simulink model "TeamA_PAsqualo1"  (R2020a)
settings: Solver=VariableStepAuto  StartTime=0.0  StopTime=stop_time  FixedStep=0.05  RelTol=1e-3
InitFcn:
  | main_init
values from neighbouring files (symbols this model uses):
  a1 = rho * D^4 * alpha1    (= 0.000388302366464)    [data_current.m]    (also in main_init.m)
  a2 = -rho * D^3 * alpha2 * (1 - omega)    (= 0.0037030698432)    [data_current.m]    (also in main_init.m)
  ag = [Ax Ay Az]'    [init_modello.m]
  alpha1 = 0.0113    [data_current.m]    (also in main_init.m)
  alpha2 = -0.0091    [data_current.m]    (also in main_init.m)
  areaOfInterestCorner = [42.317744;10.915136; 0]    [init_controllo.m]    (also in missionA.m = [42.317744)
  bg = [Bx By Bz]'    [init_modello.m]
  cd_pitch = 0.7    [init_modello.m]
  cd_roll = 0.04    [init_modello.m]
  cd_x = 0.4    [init_modello.m]
  cd_y = 1    [init_modello.m]
  cd_yaw = 0.7    [init_modello.m]
  cd_z = 1    [init_modello.m]
  cg = [Cx Cy Cz]'    [init_modello.m]
  D = 0.076    [data_current.m]    (also in main_init.m)
  dead_zone_limit = 31.5    [data_current.m]    (also in main_init.m)
  dg = [Dx Dy Dz]'    [init_modello.m]
  eg = [Ex Ey Ez]'    [init_modello.m]
  fg = [Fx Fy Fz]'    [init_modello.m]
  g = 9.81    [init_modello.m]
  galleggiamento = 66.5386    [init_controllo.m]
  gg = [Gx Gy Gz]'    [init_modello.m]
  H0 = 0    [init_modello.m]
  init_position = [pointP(1),pointP(2),0.15,0,0,deg2rad(angle)]'    [appunti.m]    (also in init_modello.m = [pointP(1),pointP(2),0.15,0,0,deg2rad(alpha)]')
  init_velocity = [0 0 0 0 0 0]'    [init_modello.m]
  initial_state_cov = blkdiag(diag(cov_gps(1,1:2)), cov_depth*eye(n_state_filter-2))    [init_navigazione.m]
  Ixx = 0.93304097392    [init_modello.m]
  Ixy = 0    [init_modello.m]
  Ixz = 0    [init_modello.m]
  Iyy = 25.58745481378    (= 25.5874548138)    [init_modello.m]
  Iyz = 0    [init_modello.m]
  Izz = 25.58745481378    (= 25.5874548138)    [init_modello.m]
  K_i_heave_div = 20    [init_controllo.m]
  K_i_heave_pos = 1    [init_controllo.m]
  K_i_heave_surf = 20    [init_controllo.m]
  K_i_heave_trans = 5    [init_controllo.m]
  K_i_heave_turn = 5    [init_controllo.m]
  K_i_pitch_div = 0    [init_controllo.m]
  K_i_pitch_pos = 0.1*0    (= 0)    [init_controllo.m]
  K_i_pitch_surf = 0    [init_controllo.m]
  K_i_pitch_trans = 0    [init_controllo.m]
  K_i_pitch_turn = 0    [init_controllo.m]
  K_i_roll_div = 0    [init_controllo.m]
  K_i_roll_pos = 0.1*0    (= 0)    [init_controllo.m]
  K_i_roll_surf = 1    [init_controllo.m]
  K_i_roll_trans = 0    [init_controllo.m]
  K_i_roll_turn = 0    [init_controllo.m]
  K_i_surge_div = 3    [init_controllo.m]
  K_i_surge_pos = 0.1679*30    (= 5.037)    [init_controllo.m]
  K_i_surge_surf = 3    [init_controllo.m]
  K_i_surge_trans = 0.1679*15    (= 2.5185)    [init_controllo.m]
  K_i_surge_turn = 0.1679*60    (= 10.074)    [init_controllo.m]
  K_i_sway_div = 6    [init_controllo.m]
  K_i_sway_pos = 5    [init_controllo.m]
  K_i_sway_surf = 3    [init_controllo.m]
  K_i_sway_trans = 2    [init_controllo.m]
  K_i_sway_turn = 50    [init_controllo.m]
  K_i_yaw_div = 0    [init_controllo.m]
  K_i_yaw_pos = 1    [init_controllo.m]
  K_i_yaw_surf = 0    [init_controllo.m]
  K_i_yaw_trans = 20    [init_controllo.m]
  K_i_yaw_turn = 3    [init_controllo.m]
  K_p_heave_div = 200    [init_controllo.m]
  K_p_heave_pos = 320    [init_controllo.m]
  K_p_heave_surf = 200    [init_controllo.m]
  K_p_heave_trans = 170    [init_controllo.m]
  K_p_heave_turn = 170    [init_controllo.m]
  K_p_phi_div = 0.15    [init_controllo.m]
  K_p_phi_pos = 1*0.1    (= 0.1)    [init_controllo.m]
  K_p_phi_surf = 0.15    [init_controllo.m]
  K_p_phi_trans = 0.1    [init_controllo.m]
  K_p_phi_turn = 0.1    [init_controllo.m]
  K_p_pitch_div = 50    [init_controllo.m]
  K_p_pitch_pos = 25    [init_controllo.m]
  K_p_pitch_surf = 50    [init_controllo.m]
  K_p_pitch_trans = 25    [init_controllo.m]
  K_p_pitch_turn = 25    [init_controllo.m]
  K_p_psi_div = 0.3    [init_controllo.m]
  K_p_psi_pos = 0.25    [init_controllo.m]
  K_p_psi_surf = 0.3    [init_controllo.m]
  K_p_psi_trans = 0.2    [init_controllo.m]
  K_p_roll_div = 10    [init_controllo.m]
  K_p_roll_pos = 0.1*40    (= 4)    [init_controllo.m]
  K_p_roll_surf = 10    [init_controllo.m]
  K_p_roll_trans = 0.1*40    (= 4)    [init_controllo.m]
  K_p_roll_turn = 4    [init_controllo.m]
  K_p_surge_div = 80    [init_controllo.m]
  K_p_surge_pos = 13.7782*2.5    (= 34.4455)    [init_controllo.m]
  K_p_surge_surf = 80    [init_controllo.m]
  K_p_surge_trans = 20    [init_controllo.m]
  K_p_surge_turn = 150    [init_controllo.m]
  K_p_sway_div = 100    [init_controllo.m]
  K_p_sway_pos = 90    [init_controllo.m]
  K_p_sway_surf = 80    [init_controllo.m]
  K_p_sway_trans = 80    [init_controllo.m]
  K_p_sway_turn = 200    [init_controllo.m]
  K_p_th_div = 0.3    [init_controllo.m]
  K_p_th_pos = 0.1    [init_controllo.m]
  K_p_th_surf = 0.3    [init_controllo.m]
  K_p_th_trans = 0.1    [init_controllo.m]
  K_p_th_turn = 0.1    [init_controllo.m]
  K_p_x_div = 0.12    [init_controllo.m]
  K_p_x_pos = 0.12    [init_controllo.m]
  K_p_x_surf = 0.12    [init_controllo.m]
  K_p_y_div = 0.6    [init_controllo.m]
  K_p_y_pos = 0.34    [init_controllo.m]
  K_p_y_surf = 0.1    [init_controllo.m]
  K_p_y_trans = 0.3    [init_controllo.m]
  K_p_y_turn = 0.3    [init_controllo.m]
  K_p_yaw_div = 70    [init_controllo.m]
  K_p_yaw_pos = 20    [init_controllo.m]
  K_p_yaw_surf = 70    [init_controllo.m]
  K_p_yaw_trans = 160    [init_controllo.m]
  K_p_yaw_turn = 60    [init_controllo.m]
  K_p_z_div = 0.35    [init_controllo.m]
  K_p_z_pos = 0.2    [init_controllo.m]
  K_p_z_surf = 0.35    [init_controllo.m]
  K_p_z_trans = 0.10    (= 0.1)    [init_controllo.m]
  K_p_z_turn = 0.1    [init_controllo.m]
  Kadd = 0    [init_modello.m]
  ... (+61 more)
undefined symbols (not defined in the file or in its folder): DiscIntNeverNeededParam, initial_state
libraries: simulink x4, vrlib x1
(part 5 of 6)

== stateflow chart TeamA_PAsqualo1/Mission Supervisor Def/State Management ==
  state Movements [parallel]
    settings: executionOrder=1
    state End [function]
    state positioning
      entry:
      current_state(1:5) = [1 0 0 0 0];
      orBene = 0; %ENGLISH
      velNull = 0;
      fromFirstPos = 0;
      during:
      if ~missionEnd %Mission just started
      if ~checkOr([0,0,orDes],orient,errOrPos) && ~orBene
      pos_ref = pointP;
      orient_ref = [0,0,orDes];
      vel_ref = [0,0,0,0,0,0];
      else %Properly oriented
      orBene=1;
      pos_ref = pointA;
      orient_ref = [0,0,orDes];
      vel_ref = velPos;
      end
      else %Mission successfully completed
      pos_ref = pointP;
      orient_ref = [0,0, orDesRit];
      vel_ref = velPos;
      end
    state diving
      entry:
      current_state(1:5) = [0 1 0 0 0];
      velNull = 0;
      during:
      %First, the vehicle stops and stabilizes in point A
      if ~(checkPos(pointA,pos, errSphere) && checkOr([0,0,orDes],orient,errOrPos) ...
      && checkVel(zeros(1,6),[vel(1),vel(2),vel(3),0,0,0],errVelDiv)) && ~velNull
      pos_ref = pointA;
      orient_ref = [0,0,orDes];
      vel_ref = zeros(1,6);
      else
      % Then it starts the descent
      velNull = 1;
      pos_ref = [pointA(1),pointA(2), averageDepth - altitude];
      orient_ref = orientA;
      if (pos_ref(3) - pos(3) > endDiv)
      vel_ref = velSub;
      else %In the last meters
      vel_ref = velRidSub;
      end
      end
    note: Transition activated when the vehicle has returned to Point P after a successful mission
    note: Transition activated when the vehicle is properly oriented in point A
    note: Transition activated when the vehicle has returned to the surface
    state surfacing
      entry:
      current_state(1:5) = [0 0 0 0 1];
      velNull = 0;
      during:
      if wall || current_state(8) %Mission aborted because of obstacles or failures
      pos_ref = [pos(1), pos(2), 0.15];
      vel_ref = velSurf;
      else
      %First the vehicle stops and stabilizes at the end of the trajectory
      if ~checkVel(zeros(1,6),[vel(1),vel(2),vel(3),0,0,0],errVelSurf) && ~velNull
      pos_ref = trWP(nWPTran,:,nTran);
      orient_ref = [0,0,orDesRit];
      vel_ref = zeros(1,6);
      else
      %Then it starts the ascent
      velNull = 1;
      ptSup = trWP(nWPTran,:,nTran);
      pos_ref = [ptSup(1),ptSup(2),0.15];
      orient_ref = [0,0,orDesRit];
      vel_ref = velSurf;
      end
      end
    note: Transition activated when the vehicle is underwater
        | at desired position and orientation
    note: Transition activated when the vehicle has properly
        | arrived at the end of the trajectory
    state turn
      entry:
      current_state(1:5) = [0 0 0 1 0];
      state ReferencePoints
        note: References provided during the turn
        note: Last references
        note: Even numbered transects
        note: Odd numbered transects
        (default) -> (junction 728)
        (junction 728) -> (junction 736) [order 2] : {pos_ref = turnWP(nWPTurn,:,page);
            | orient_ref = deg2rad(turnRef(nWPTurn,:,page));}
        (junction 728) -> (junction 733) [order 1] : [time+1<=nWPTurn]
            | {pos_ref = turnWP(time+1,:,page);
            | orient_ref = deg2rad(turnRef(time+1,:,page));}
        (junction 736) -> (junction 733)
        (junction 733) -> (junction 738) [order 1] : [mod(page,2) == 0]
            | {vel_ref = [0.2 0 0 0 0 -rot*0.2/(lineSpaceBetweenTransects/2)];}
        (junction 733) -> (junction 731) [order 2] : {vel_ref = [0.2 0 0 0 0 rot*0.2/(lineSpaceBetweenTransects/2)];}
      ReferencePoints -> ReferencePoints
      (default) -> ReferencePoints
    state transect
      entry:
      current_state(1:5) = [0 0 1 0 0];
      ptx = trWP(wpTR,:,page);
      pos_ref = [ptx(1),ptx(2),pos(3)-(altitude-FLS_down)];
      if mod(page,2) == 0 %Even numbered transects
      orient_ref = orPari;
      else
      orient_ref = orDispari; %Odd numbered transects
      end
      vel_ref = velTran;
      state Disaligned
        note: If emergency WPs have not been generated
        note: Last WPs
        note: Emergency WPs already generated
        note: Emergency WPs generations
        note: Providing references
        note: Odd numbered turns
        note: Even numbered turns
        note: If current WP has been reached
        note: Last emergency WP reached
        (default) -> (junction 490)
        (junction 490) -> (junction 207) : {sizeEmerg = size(wpEmerg);}
        (junction 207) -> (junction 674) [order 1] : [~all(sizeEmerg)]
        (junction 674) -> (junction 681) [order 2] : {wpTR = nWPTran;}
        (junction 207) -> (junction 210) [order 2]
        (junction 674) -> (junction 681) [order 1] : [wpTR + 2 <= nWPTran]
            | {wpTR = wpTR+2;}
        (junction 681) -> (junction 210) : {wpEmerg = currentSwingWaypoints(trWP(wpTR,:,page),pos,distEmerg);}
        (junction 210) -> (junction 396) : {ptx = wpEmerg(idxEmerg,1:3);
            | pos_ref = [ptx(1),ptx(2),pos(3)-(altitude-FLS_down)];
            | vel_ref = vEmergTran;}
        (junction 396) -> (junction 225) [order 1] : [mod(page,2) == 0]
            | {orient_ref = orPari;}
        (junction 396) -> (junction 225) [order 2] : {orient_ref =orDispari;}
        (junction 225) -> (junction 259) [order 2]
        (junction 225) -> (junction 213) [order 1] : [checkPos(pos,pos_ref,errPosWPTrans) &&...
            | checkOr(orient,orient_ref,errOrWPTrans)]
        (junction 213) -> (junction 215) [order 1] : [idxEmerg == size(wpEmerg,1)]
            | {idxEmerg = 1; current_state(6) = 0;}
        (junction 213) -> (junction 215) [order 2] : {idxEmerg = idxEmerg + 1;}
      state Aligned
        note: For the last WPs
        note: If current WP has been reached
        note: Next WP index
        note: Providing references
        note: Even numbered transects
        note: Odd numbered transects
        note: Last WPs
        (default) -> (junction 203)
        (junction 203) -> (junction 754) [order 2] : {error=errPosTransLast;}
        (junction 203) -> (junction 754) [order 1] : [wpTR<=nWPTran-2]
            | {error=errPosTrans;}
        (junction 754) -> (junction 219) [order 2]
        (junction 754) -> (junction 663) [order 1] : [checkPos(pos_ref,pos,error) && ...
            | checkOr(orient_ref,orient,errOrTrans)]
        (junction 663) -> (junction 219) : [wpTR+1 <= nWPTran]
            | {wpTR = wpTR + 1;}
        (junction 219) -> (junction 393) : {wpEmerg =  [];
            | ptx = trWP(wpTR,:,page);
            | pos_ref = [ptx(1),ptx(2),pos(3)-(altitude-FLS_down)];}
        (junction 393) -> (junction 222) [order 1] : [mod(page,2) == 0]
            | {orient_ref = orPari;}
        (junction 393) -> (junction 222) [order 2] : {orient_ref = orDispari;}
        (junction 222) -> (junction 227) [order 1] : [wpTR > nWPTran - 2]
            | {vel_ref = velRid;}
        (junction 222) -> (junction 227) [order 2] : {vel_ref = velTran;}
      note: Vehicle has realigned
      note: Misalign detected
      Aligned -> Aligned [order 2]
      Disaligned -> Disaligned [order 2]
      (default) -> Aligned
      Disaligned -> Aligned [order 1] : [~current_state(6)]
      Aligned -> Disaligned [order 1] : [current_state(6)]
    note: Transition activated when all the turn references
        | have been provided to the Control block
    note: To try to have good enough performances in extreme cases
    note: Transition activated when the vehicle has travelled a complete transect
    (default) -> positioning : {missionEnd = 0;}
    positioning -> positioning [order 1] : [missionEnd && checkPos(pointP,pos,errPosPos/2)]
        | {End();}
    positioning -> diving [order 2] : [checkPos(pointA,pos,errPosPos) && checkOr([0,0,orDes],orient,errOrPos)]
    positioning -> surfacing [order 3] : [wall || current_state(8)]
        | {fromFirstPos = 1;}
    diving -> surfacing [order 2] : [wall || current_state(8)]
    diving -> transect [order 1] : [checkPos3([pointA(1),pointA(2), pos(3)-(altitude-FLS_down)],pos,errPosDiv) ...
        | && checkOr(orientA,orient,errOrDiv)]
    surfacing -> positioning [order 1] : [checkPos3([ptSup(1),ptSup(2),0.15],pos,errPosSurf) && ...
        | checkOr([0,0,orDesRit],orient,errOrSurf) && checkVel(zeros(1,6),vel,errVelSurf)...
        | && ~fromFirstPos]
        | {missionEnd = 1;}
    surfacing -> surfacing [order 2] : [wall && ...
        | checkPos3([pos(1),pos(2),0.15],pos_ref, errPosSurf)]
        | {End();}
    transect -> surfacing [order 1] : [wall || current_state(8)]
    turn -> surfacing [order 2] : [wall || current_state(8)]
    transect -> surfacing [order 2] : [(checkPos(trWP(nWPTran,:,nTran),pos, errPosTrans) &&...
        | checkOr(orient_ref,orient,errOrTrans))]
    (junction 872) -> transect [order 2] : {wpTR = 1;}
    turn -> (junction 872) [order 1] : [time+1 == nWPTurn]
        | {page = page + 1;}
    (junction 872) -> transect [order 1] : [cruiseSpeed>=1.5 && lineSpaceBetweenTransects<4]
        | {wpTR = 2;}
    transect -> turn [order 3] : [checkPos(trWP(nWPTran,:,page),pos, errPosTransLast) && checkOr(orient_ref,orient,errOrTrans)]
        | {wpTU=1;}
  state Issues_management [parallel]
    entry:
    points=[];
    profs=[];
    settings: executionOrder=2
    state Free
      entry:
      current_state(6:8) = 0;
      during:
      %During positioning and surfacing
      if current_state(1) || current_state(5)
      pos_ref(3) = 0.15;
      else
      %During the other states, the depth reference
      %will be overwritten by this
      if abs(altitude - FLS_down)>=minGap
      pos_ref(3)= pos(3) - (altitude - FLS_down);
      else
      pos_ref(3) = pos(3);
      end
      end
    state Issue_found
      state obstacle %checks for walls or obstacles [parallel]
        entry,during:
        distFront = FLS_front*cos(deg2rad(theta_f));
        distDown = FLS_front*sin(deg2rad(theta_f));
        oDeg= rad2deg(orient);
        nedFLS = fix2LocalNED(oDeg(1),oDeg(2),oDeg(3))'*[distFront;0;distDown];
        pointProf = pos(3) - (altitude-FLS_down) - (FLS_down-nedFLS(3));
        pointApp = calcPoint(pos,oDeg,nedFLS(1));
        nedAxis = (fix2LocalNED(oDeg(1),oDeg(2),oDeg(3))'*[semix; semiy; semiz])';
        settings: executionOrder=3
        note: There are some obstacles already detected
        note: No obstacles detected, yet
        note: After some evaluation on the measure received by the frontal FLS,
            | this states is based on the ratio between the altitude gap to overcome
            | and estimated distance needed to actually change the vehicle depth
            | position to the new value.
            | If this ratio is greater than the one calculated based on data received
            | from the Control block, the obstacle is considered as a wall impeding
            | further advancement of the vehicle and the mission is aborted.
            | This is because it cannot be ensured that the reference depth above
            | the obstacle will be reached and in case of a steep ridge the vehicle
            | could crash with it and be damaged.
        note: If the vehicle is approaching the nearest obstacle
        note: If the vehicle has reached the nearest obstacle
        note: Wall detected, based on the ratio calculated
        note: There are other obstacles to be overtook
        note: If the obstacle cannot be ignored, based on its dimensions
        note: Deciding if obstacle can be ignored
        note: If the gap between the last seen obstacle and the newly detected one
            | is such that the vehicle wouldn't be able to overcome one after another,
            | the last seen obstacle is ignored and the vehicle will move above the
            | newly detected one; this will cause an overshoot of the desired altitude
            | above the last seen obstacle but will ensure further mission advancements
        (default) -> (junction 563)
        (junction 563) -> (junction 800) [order 1] : [~current_state(3)]
            | {points = [];profs=[];}
        (junction 563) -> (junction 575) [order 3] : [~all(size(points))]
        (junction 563) -> (junction 565) [order 2] : [all(size(points))]
            | {distObsVeh = distance(pos+nedAxis,points(1,:));
            | punto = points(1,:);}
        (junction 565) -> (junction 789) [order 2] : [distObsVeh>(abs(pos(3)-profs(1))...
            | /maxRatio + safeMargin)]
        (junction 565) -> (junction 567) [order 1] : [distObsVeh<=(abs(pos(3)-profs(1))/maxRatio + safeMargin)]
            | {pos_ref(3) = profs(1);}
        (junction 575) -> (junction 573)
        (junction 567) -> (junction 791)
        (junction 789) -> (junction 791)
        (junction 791) -> (junction 573) [order 2]
        (junction 791) -> (junction 573) [order 1] : [checkPos([punto(1),punto(2),profs(1)],pos,errPosPos)]
            | {points  = points(2:end,:);}
        (junction 573) -> (junction 578) [order 1] : [abs(pos(3) - pointProf)/(distFront+nedAxis(1)) > maxRatio]
            | {current_state(7) = 1;wall = 1;}
        (junction 573) -> (junction 605) [order 3]
        (junction 573) -> (junction 580) [order 2] : [abs(pos(3) - pointProf)/(distFront+nedAxis(1)) <= maxRatio]
        (junction 580) -> (junction 582) [order 1] : [all(size(points))]
            | {distObs = distance(points(end,:),pointApp);}
        (junction 580) -> (junction 794) [order 2] : [~all(size(points))]
        (junction 794) -> (junction 796) [order 2]
        (junction 794) -> (junction 586) [order 1] : [abs(pos(3)-pointProf)>=minGap]
            | {distObsVeh=distance(pos,pointApp);}
        (junction 582) -> (junction 785) [order 2]
        (junction 582) -> (junction 584) [order 1] : [abs(profs(end)-pointProf)>=minGap]
        (junction 586) -> (junction 787) [order 2]
        (junction 586) -> (junction 588) [order 1] : [distObsVeh>=minDist+nedAxis(1)]
            | {points = addP(points,pointApp);}
        (junction 584) -> (junction 590) [order 1] : [distObs < minDist || abs(profs(end)-pointProf)/distObs > maxRatio]
            | {points = points(1:end-1,:);}
        (junction 584) -> (junction 592) [order 2]
        (junction 590) -> (junction 592)
        (junction 592) -> (junction 595) : {points=addP(points,pointApp);}
      state warning %disalignment [parallel]
        during:
        %Disalignment check activated only during the transect
        if current_state(3)
        disalignOP;
        end
        if current_state(1) || current_state(5)
        pos_ref(3) = 0.15;
        else
        if abs(altitude - FLS_down)>=minGap
        pos_ref(3)= pos(3) - (altitude - FLS_down);
        else
        pos_ref(3) = pos(3);
        end
        end
        settings: executionOrder=1
      state abort %vehicle failures [parallel]
        entry:
        inactivity = 1;
        during:
        checkFailure;
        settings: executionOrder=2
      state disalignOP [function]
        note: The alignment check is different depending whether
            | the vehicle is at the end of the transect or not
        (default) -> (junction 696)
        (junction 696) -> (junction 700) [order 1] : [current_state(3) && wpTR >=2 &&...
            | retta(pos,trWP(1,:,page),trWP(nWPTran,:,page))>=offset]
            | {current_state(6) = 1;}
        (junction 696) -> (junction 747) [order 2] : [current_state(3) && wpTR>nWPTran-2 ...
            | && retta(pos,trWP(1,:,page),trWP(nWPTran,:,page))>=offsetLast]
            | {current_state(6) = 1;}
        (junction 696) -> (junction 780) [order 3]
      state checkFailure [function]
        note: Checks if the motors are failing
        (default) -> (junction 108)
        (junction 108) -> (junction 109) : [vel(1:3) == [0 0 0]]
            | {inactivity = inactivity + 1;}
        (junction 109) -> (junction 114) : [mod(inactivity,1000) == 0]
            | {current_state(8) = 1;}
    state rit = check [function]
      note: Check for any problem
      (default) -> (junction 122)
      (junction 122) -> (junction 479) [order 2] : {rit = 0;}
      (junction 122) -> (junction 124) [order 1] : [(current_state(3) && wpTR >=2 &&...
          | retta(pos,trWP(1,:,page),trWP(nWPTran,:,page))>=offset) ||...
          | current_state(3) && wpTR>nWPTran-2 ...
          | && retta(pos,trWP(1,:,page),trWP(nWPTran,:,page))>=offsetLast ||...
          |  all(size(points)) ]
          | {rit = 1;}
    (default) -> Free
    Free -> Issue_found : [check]
    Issue_found -> Free : [~check]
  data: puntoDes function_input; puntoCorr function_input; dist function_input; M function_output; ang constant double =angle; vRef function_input; vAct function_input; vErr function_input; okVel function_output; oRef function_input; oAct function_input; oErr function_input; okOr function_output; pRef function_input; pAct function_input; pErr function_input; okPos function_output; pRef function_input; pAct function_input; pErr function_input; okPos function_output; lista function_input; p function_input; pointrit function_output; distPR function_output; position function_input; p1 function_input; p2 function_input; phi function_input; theta function_input; rotation function_output; psi function_input; pRef function_input; pAct function_input; pErr function_input; okPos function_output; p function_input; o function_input; pt function_output; d function_input; p1 function_input; p2 function_input; valDist function_output; distPR function_output; position function_input; p1 function_input; p2 function_input; rit function_output; current_state output size=[1, 8] =[0 0 0 0 0 0 0 0]; pos_ref output =pointP; orient_ref output size=[1 3] =[0 0 deg2rad(angle)]; pos input; orient input; vel input; FLS_front input; FLS_down input; time input; vel_ref output =[0 0 0 0 0 0]; orientA parameter; velPos parameter; velSub parameter; velSurf parameter; velTran parameter; wpEmerg local size=[200 3] =zeros(200,3); altitude parameter; averageDepth parameter; nTran parameter; nWPTran parameter; nWPTurn parameter; pointP parameter; trWP parameter; turnWP parameter; velRid parameter; idxEmerg local =1; missionEnd local =0; endDiv parameter; turnRef parameter; velRidSub parameter; errOrDiv parameter; errOrSurf parameter; errOrTrans parameter; errOrWPTrans parameter; errPosDiv parameter; errPosSurf parameter; errPosTrans parameter; errPosWPTrans parameter; errVelDiv parameter; errVelSurf parameter; inactivity local =1; errOrPos parameter; errPosPos parameter; vEmergTran parameter; offset parameter; sizeEmerg local size=[1,2] =[0 0]; distEmerg parameter; pointA parameter; wpTR local =1; wpTU local =1; page local =1; maxRatio parameter; minDist parameter; minGap parameter; profs local size=[1 20] =zeros(1,20); semix parameter; semiy parameter double; semiz parameter; theta_f parameter; distObsVeh local size=1 =0; distDown local size=1 =0; distFront local size=1 =0; nedAxis local size=[1,3] =zeros(1,3); nedFLS local; pointApp local size=[1,2] =zeros(1,2); pointProf local size=[1 1] =0; distObs local size=1 =0; safeMargin parameter; orDes parameter; orBene local; velNull local; errSphere parameter; ptx local =[0 0 0]; lineSpaceBetweenTransects parameter; ptSup local size=[1 3] =zeros(1,3); orDesRit parameter; orDispari parameter; orPari parameter; fromFirstPos local; wall local =0; rot parameter; errPosTransLast parameter; error local; offsetLast parameter; punto local size=[1 3]; oDeg local; points local size=[20,2] =[]; cruiseSpeed parameter
  function M = currentSwingWaypoints(puntoDes,puntoCorr,dist):
    | function M = currentSwingWaypoints(puntoDes,puntoCorr,dist)
    | %CURRENTSWINGWAYPOINTS generates additional waypoints to be used when the
    | % vehicle misaligns from the desired trajectory
    | %
    | %   -puntoDes: desired return point onto the trajectory; 1x3 [m m m]
    | %   -puntoCorr: estimated current location; 1x3 [m m m]
    | %   -dist: distance between waypoints in the direction of realignment; [m]
    | 
    |     distN = puntoCorr(1) - puntoDes(1); %Distance from starting and final point onto the North axis
    |     distE = puntoCorr(2) - puntoDes(2); %Distance from starting and final point onto the East axis
    | 
    |     %Number of waypoints to generate
    |     p = floor(abs(distE)/dist);
    |     
    |     deltaE = distE/p; %Distance between two waypoints onto the North axis
    |     deltaN = distN/p; %Distance between two waypoints onto the East axis
    |    
    |     matrix = zeros(p-1,3);
    |    
    |     %Ending at p-1 because the last additional waypoint corresponds to
    |     %"standard" waypoint onto the trajectory
    |     for i = 1:p-1
    |         %Waypoint generation
    |         waypoint = puntoCorr - i * [deltaN deltaE 0];
    |         waypoint(3) = puntoDes(3);
    |         matrix(i,:) = waypoint;
    |     end
    |     
    |     M = matrix;   
    |    
    | end
  function okVel = checkVel(vRef,vAct,vErr):
    | function okVel = checkVel(vRef,vAct,vErr)
    | %CHECKVEL checks that the current and the desired velocities are "almost"
    | %the same, considering an allowed tolerance
    | %
    | %   -vRef: desired velocity
    | %   -vAct: current velocity
    | %   -vErr: allowed tolerance
    | 
    |     okVel = all(abs(vRef - vAct) <= vErr);
    | end
  function okOr = checkOr(oRef,oAct,oErr):
    | function okOr = checkOr(oRef,oAct,oErr)
    | %CHECKOR checks that the current ant the desired orientations are the same,
    | %considering an allowed tolerance
    | %
    | %   -oRef: desired orientation
    | %   -oAct: current orientation
    | %   -oErr: allowed tolerance
    | 
    |     okOr = all(abs(oRef - oAct) <= oErr);
    | end
  function okPos = checkPos(pRef,pAct,pErr):
    | function okPos = checkPos(pRef,pAct,pErr)
    | %CHECKPOS checks that the current and the desired positions are "almost"
    | %the same, considering an allowed tolerance; this function does not
    | %contemplates the depth reference
    | %
    | %   -pRef: desired position
    | %   -pAct: current position
    | %   -pErr: allowed tolerance
    | 
    |     okPos = all(abs(pRef(1:2) - pAct(1:2))  <= pErr(1:2));
    | end
  function okPos = checkPos3(pRef,pAct,pErr):
    | function okPos = checkPos3(pRef,pAct,pErr)
    | %CHECKPOS3 checks that the current and the desired positions are "almost"
    | %the same, considering an allowed tolerance; this function also
    | %contemplates the depth reference
    | %
    | %   -pRef: desired position
    | %   -pAct: current position
    | %   -pErr: allowed tolerance
    | 
    |     okPos = all(abs(pRef - pAct)  <= pErr);
    | end
  function pointrit = addP(lista,p):
    | function pointrit = addP(lista,p)
    | %ADDP ensure that the new point refering to an obstacle is properly added
    | %to the current obstacle list, avoiding evaluation problems
    | %
    | %   -lista: current list
    | %   -p: point to be added
    | 
    |     if ~all(size(lista))
    |         app = [];
    |         pointrit = cat(1,app,p);
    |     else
    |         pointrit = cat(1,lista,p);
    |     end
    | end
  function distPR = retta(position,p1,p2):
    | function distPR = retta(position,p1,p2)
    | %RETTA returns the distance between the specified point "position" and the
    | %straight line passing through p1 and p2
    | 
    |     m = p2-p1;
    |     coeff=m(2)/m(1); %Angular coefficient
    |     distPR = abs(position(2)-(coeff*(position(1)-p1(1))+p1(2)))/sqrt(1+coeff^2);
    |     %y-y1 = m*(x-x1) -> y = m*(x-x1)+y1
    | end
  function rotation = fix2LocalNED(phi, theta, psi):
    | function rotation = fix2LocalNED(phi, theta, psi)
    | %FIX2LOCALNED generates the matrix describing the RPY rotation between the
    | %NED reference system and the reference system aligned with the vehicle
    | %axis
    | %
    | %   -phi: x axis angle; [°]
    | %   -theta: y axis angle; [°]
    | %   -psi: z axis angle; [°]
    | 
    |     phirad = deg2rad(phi);
    |     cr = cos(phirad);
    |     sr = sin(phirad);
    | 
    |     thetarad = deg2rad(theta);
    |     cp = cos(thetarad);
    |     sp = sin(thetarad);
    | 
    |     psirad = deg2rad(psi);
    |     cy = cos(psirad);
    |     sy = sin(psirad);
    | 
    |     rotx = [[1 0 0];
    |             [0 cr sr];
    |             [0 -sr cr]];
    | 
    |     roty = [[cp 0 -sp];
    |             [0 1 0];
    |             [sp 0 cp]];
    | 
    |     rotz = [[cy sy 0];
    |             [-sy cy 0];
    |             [0 0 1]];
    | 
    |     rotation = rotx*roty*rotz;
    | 
    | end
  function okPos = checkPos(pRef,pAct,pErr):
    | function okPos = checkPos(pRef,pAct,pErr)
    | %CHECKPOS checks that the current and the desired positions are "almost"
    | %the same, considering an allowed tolerance; this function does not
    | %contemplates the depth reference
    | %
    | %   -pRef: desired position
    | %   -pAct: current position
    | %   -pErr: allowed tolerance
    | 
    |     okPos = all(abs(pRef(1:2) - pAct(1:2))  <= pErr(1:2));
    | end
  function pt = calcPoint(p,o,d):
    | function pt = calcPoint(p,o,d)
    | %CALCPOINT calculates the NED coordinates of the point at distance d along
    | %the surge axi of the vehicle
    | 
    |     nedDist = fix2LocalNED(o(1),o(2),o(3))'*[d; 0; 0];
    |     pt = [p(1) p(2)] + [nedDist(1) nedDist(2)];
    |     
    | end
  function valDist = distance(p1,p2):
    | function valDist = distance(p1,p2)
    | %DISTANE calculates the distance between p1 and p2 in the XY plane
    |     valDist = sqrt((p1(1)-p2(1))^2 + (p1(2)-p2(2))^2);
    | end
  function distPR = retta(position,p1,p2):
    | function distPR = retta(position,p1,p2)
    | %RETTA returns the distance between the specified point "position" and the
    | %straight line passing through p1 and p2
    | 
    |     m = p2-p1;
    |     coeff=m(2)/m(1); %Angular coefficient
    |     distPR = abs(position(2)-(coeff*(position(1)-p1(1))+p1(2)))/sqrt(1+coeff^2);
    |     %y-y1 = m*(x-x1) -> y = m*(x-x1)+y1
    | end

== matlab function TeamA_PAsqualo1/Mission Supervisor Def/Trasf. to LLD ==
  data: posArg input; pos output; areaOfInterestCorner parameter
function pos = NED2LLD(posArg,areaOfInterestCorner)
    coder.extrinsic('evalin','wgs84Ellipsoid','ned2geodetic');
    pos = zeros(1,3);
    pos1 = 0;
    pos2 = 0;
    pos3 = 0;
    [pos1, pos2, pos3] = ned2geodetic(posArg(1), posArg(2), posArg(3),areaOfInterestCorner(1), areaOfInterestCorner(2), 0,wgs84Ellipsoid);
    pos = [pos1, pos2, posArg(3)];%-posArg(3)];
end

== matlab function TeamA_PAsqualo1/Mission Supervisor Def/Trasf. to NED ==
  data: posArg input; pos output; areaOfInterestCorner parameter
function pos = LLD2NED(posArg,areaOfInterestCorner)
    coder.extrinsic('evalin','wgs84Ellipsoid','geodetic2ned');
    pos = zeros(1,3);
    pos1 = 0;
    pos2 = 0;
    pos3 = 0;
    [pos1, pos2, pos3] = geodetic2ned(posArg(1), posArg(2), posArg(3),areaOfInterestCorner(1), areaOfInterestCorner(2), 0,wgs84Ellipsoid);
    pos = [pos1, pos2, posArg(3)];
end

== matlab function TeamA_PAsqualo1/Controller/abort mission/abort mission ==
  data: enable input; abort output size=[6 1]; ref input; est_meas input
function abort = fcn(enable, ref, est_meas)
tau = zeros(6,1);
abort = zeros(6,1);
if enable == 1
    abort = tau;
else
    abort = tau;
end
end

== matlab function TeamA_PAsqualo1/Controller/compute n_des ==
  settings: updateMethod=DISCRETE  sampleTime=0.1
  data: enable input size=6; n_des output size=[7 1]; tau_pos input size=6; tau_div input size=6; tau_trans input size=6; tau_turn input size=6; tau_surf input size=6; abort input size=6
function n_des = fcn(enable, tau_pos, tau_div, tau_trans, tau_turn, tau_surf, abort)
j = 0;
tau = zeros(6,1);
for i=1:1:length(enable)
    if enable(i) == 1
        j = i;
    end
end
if j == 1
    tau = tau_pos;
end
if j == 2
    tau = tau_div;
end
if j == 3
    tau = tau_trans;
end
if j == 4
    tau = tau_turn;
end
if j == 5
    tau = tau_surf;
end
if j == 6
    tau = abort;
end
% Definisco la matrice di allocazione ai trust B
p_1 = [0.6  0.15 0.005]';
p_2 = [0.6 -0.15 0.005]';
p_3 = [0  0.2 0]';
p_4 = [0 -0.2 0]';
p_5 = [-1.2  0  0.005]';
p_6 = [-0.9  0  0]';
p_7 = [ 0.9  0  0]';

t_1 = [0 0 1]';
t_2 = [0 0 1]';
t_3 = [1 0 0]';
t_4 = [1 0 0]';
t_5 = [0 0 1]';
t_6 = [0 1 0]';
t_7 = [0 1 0]';

B_1 = [t_1;cross(p_1,t_1)];
B_2 = [t_2;cross(p_2,t_2)];
B_3 = [t_3;cross(p_3,t_3)];
B_4 = [t_4;cross(p_4,t_4)];
B_5 = [t_5;cross(p_5,t_5)];
B_6 = [t_6;cross(p_6,t_6)];
B_7 = [t_7;cross(p_7,t_7)];

B = [B_1 B_2 B_3 B_4 B_5 B_6 B_7];
B_pinv = pinv(B);

% Forze desiderate dei truster

T = B_pinv*tau;

% Conversione delle forze desiderate dei truster in numero di giri
b1 = 0.0003883;
u = T/b1;
offset = 31.5;   %limite della zona morta
n = zeros(7,1);
for i = 1:1:7
    n(i) = sign(u(i))*sqrt(abs(u(i)));
    n(i) = n(i) + sign(n(i))*offset;
end
n_des = n;

== matlab function TeamA_PAsqualo1/Controller/compute_if_enable ==
  settings: updateMethod=DISCRETE  sampleTime=0.1
  data: current_state input size=[8 1]; enable output size=[6 1]
function enable = fcn(current_state)
enable = zeros(6,1);
for i = 1:1:length(current_state)
    if (current_state(i) == 1 && i <= 5)
        enable(i) = 1;
    end
    if i > 5
        if (current_state(i) == 1 && i == 7)
            enable = zeros(6,1);
            enable(2) = 1;
        end
        if (current_state(i) == 1 && i == 8)
            enable = zeros(6,1);
            enable(2) = 0;
            enable(6) = 1;
        end
    end
end
end

== matlab function TeamA_PAsqualo1/Controller/diving controller/heave_controller/Heave PID controller/compute_position_errors ==
  settings: updateMethod=DISCRETE  sampleTime=0.1
  data: enable input size=1; err_pos output size=1; ref input size=[12 1]; est_state input size=[12 1]; w_des output size=1; areaOfInterestCorner parameter
function [err_pos, w_des] = fcn(enable, ref, est_state,areaOfInterestCorner)
references_NED = zeros(3,1);
est_state_NED  = zeros(3,1);
phi = est_state(4);
th  = est_state(5);
psi = est_state(6);
coder.extrinsic('evalin','wgs84Ellipsoid','geodetic2ned')    % Reference spheroid
orig = [areaOfInterestCorner(1)   areaOfInterestCorner(2)   areaOfInterestCorner(3)]'; %origine terna NED
wgs84 = wgs84Ellipsoid;
err_pos = 0;
w_des = 0;
% Cambiamento di riferimento da WGS84 a NED frame
if enable == 1
   [x_ref, y_ref, z_ref] = geodetic2ned(ref(1),ref(2),ref(3),orig(1),orig(2),orig(3),wgs84);
   references_NED = [x_ref, y_ref, z_ref]';
   [x_est, y_est, z_est] = geodetic2ned(est_state(1),est_state(2),est_state(3),orig(1),orig(2),orig(3),wgs84);
   est_state_NED  =  [x_est, y_est, z_est]';
   est_state_NED = [est_state_NED(1);est_state_NED(2);est_state(3)];
   % Calcolo errore posizione da NED a BODY frame
   err_NED  = references_NED - est_state_NED;
   R_z_psi = [cos(psi)    sin(psi)     0;
              -sin(psi)   cos(psi)     0;
                 0           0         1];
          
   R_y_th =  [cos(th)        0      -sin(th);
                 0           1         0;
              sin(th)        0       cos(th)];
       
   R_x_phi = [   1           0             0;
                 0         cos(phi)    sin(phi);
                 0        -sin(phi)    cos(phi)];
          
   R_NB = ((R_z_psi')*(R_y_th')*(R_x_phi'))';
   err_pos_BODY = R_NB * err_NED;
   offset = 0.5;  % metri di distanza dal punto desiderato
   if err_pos_BODY(3) > offset
       err_pos = 0;
       w_des   = ref(9);
   end
   if err_pos_BODY(3) <= offset
       err_pos = err_pos_BODY(3);
       w_des   = 0;
   end
else
   err_pos = 0;
   w_des   = 0;
end
end

== matlab function TeamA_PAsqualo1/Controller/diving controller/heave_controller/Heave PID controller/compute_velocity_error ==
  settings: updateMethod=DISCRETE  sampleTime=0.1
  data: enable input size=1; err_vel output size=1; v_des input size=1; est_meas input size=[12 1]
function err_vel = fcn(enable,v_des,est_meas)
if enable == 1
   err_vel =  v_des - est_meas(9);
else
    err_vel = 0;
end
end

== matlab function TeamA_PAsqualo1/Controller/diving controller/pitch_controller/Pitch PID controller/compute_orientation_errors ==
  settings: updateMethod=DISCRETE  sampleTime=0.1
  data: enable input size=1; err_orient output size=1; ref input size=[12 1]; est_state input size=[12 1]
function err_orient = fcn(enable, ref, est_state)
coder.extrinsic('wrapToPi');
err_orient = 0;
phi = est_state(4);
th  = est_state(5);
%
J_inv = [1       0          -sin(th); 
         0   cos(phi)  cos(th)*sin(phi);
         0  -sin(phi)  cos(th)*cos(phi)];
if enable == 1
   err_orient_1 = wrapToPi(J_inv*([ref(4);ref(5);ref(6)] -...
                           [est_state(4);est_state(5);est_state(6)]));
else 
   err_orient_1 = zeros(3,1);
end
err_orient = err_orient_1(2);
end

== matlab function TeamA_PAsqualo1/Controller/diving controller/pitch_controller/Pitch PID controller/compute_velocity_error ==
  settings: updateMethod=DISCRETE  sampleTime=0.1
  data: enable input size=1; err_vel output size=1; v_des input size=1; est_meas input size=[12 1]
function err_vel = fcn(enable,v_des,est_meas)
if enable == 1
   err_vel =  v_des - est_meas(11);
else
    err_vel = 0;
end
end

== matlab function TeamA_PAsqualo1/Controller/diving controller/roll_controller/Roll PID controller/compute_orientation_errors ==
  settings: updateMethod=DISCRETE  sampleTime=0.1
  data: enable input size=1; err_orient output size=1; ref input size=[12 1]; est_state input size=[12 1]
function err_orient = fcn(enable, ref, est_state)
coder.extrinsic('wrapToPi');
err_orient = 0;
phi = est_state(4);
th  = est_state(5);
%
J_inv = [1       0          -sin(th); 
         0   cos(phi)  cos(th)*sin(phi);
         0  -sin(phi)  cos(th)*cos(phi)];
if enable == 1
   err_orient_1 = wrapToPi(J_inv*([ref(4);ref(5);ref(6)] -...
                           [est_state(4);est_state(5);est_state(6)]));
else 
   err_orient_1 = zeros(3,1);
end
err_orient = err_orient_1(1);
end

== matlab function TeamA_PAsqualo1/Controller/diving controller/roll_controller/Roll PID controller/compute_velocity_error ==
  settings: updateMethod=DISCRETE  sampleTime=0.1
  data: enable input size=1; err_vel output size=1; v_des input size=1; est_meas input size=[12 1]
function err_vel = fcn(enable,v_des,est_meas)
if enable == 1
   err_vel =  v_des - est_meas(10);
else
    err_vel = 0;
end
end

== matlab function TeamA_PAsqualo1/Controller/diving controller/surge_controller/Surge PID controller/compute_position_errors ==
  settings: updateMethod=DISCRETE  sampleTime=0.1
  data: enable input size=1; err_pos output size=1; ref input size=[12 1]; est_state input size=[12 1]; areaOfInterestCorner parameter
function err_pos = fcn(enable, ref, est_state,areaOfInterestCorner)
references_NED = zeros(3,1);
est_state_NED  = zeros(3,1);
phi = est_state(4);
th  = est_state(5);
psi = est_state(6);
coder.extrinsic('evalin','wgs84Ellipsoid','geodetic2ned')    % Reference spheroid
orig = [areaOfInterestCorner(1)   areaOfInterestCorner(2)   areaOfInterestCorner(3)]'; %origine terna NED
wgs84 = wgs84Ellipsoid;
% Cambiamento di riferimento da WGS84 a NED frame
if enable == 1
   [x_ref, y_ref, z_ref] = geodetic2ned(ref(1),ref(2),ref(3),orig(1),orig(2),orig(3),wgs84);
   references_NED = [x_ref, y_ref, z_ref]';
   [x_est, y_est, z_est] = geodetic2ned(est_state(1),est_state(2),est_state(3),orig(1),orig(2),orig(3),wgs84);
   est_state_NED  =  [x_est, y_est, est_state(3)]';
   % Calcolo errore posizione da NED a BODY frame
   err_NED  = references_NED - est_state_NED;
   R_z_psi = [cos(psi)    sin(psi)     0;
              -sin(psi)   cos(psi)     0;
                 0           0         1];
          
   R_y_th =  [cos(th)        0      -sin(th);
                 0           1         0;
              sin(th)        0       cos(th)];
       
   R_x_phi = [   1           0             0;
                 0         cos(phi)    sin(phi);
                 0        -sin(phi)    cos(phi)];
          
   R_NB = ((R_z_psi')*(R_y_th')*(R_x_phi'))';
   err_pos_BODY = R_NB * err_NED;

   err_pos = err_pos_BODY(1);
else
   err_pos = 0;
end
end

== matlab function TeamA_PAsqualo1/Controller/diving controller/surge_controller/Surge PID controller/compute_velocity_error ==
  settings: updateMethod=DISCRETE  sampleTime=0.1
  data: enable input size=1; err_vel output size=1; v_des input size=1; est_meas input size=[12 1]
function err_vel = fcn(enable,v_des,est_meas)
if enable == 1
   err_vel =  v_des - est_meas(7);
else
    err_vel = 0;
end
end

== matlab function TeamA_PAsqualo1/Controller/diving controller/sway_controller/Sway PID controller/compute_position_errors ==
  settings: updateMethod=DISCRETE  sampleTime=0.1
  data: enable input size=1; err_pos output size=1; ref input size=[12 1]; est_state input size=[12 1]; areaOfInterestCorner parameter
function err_pos = fcn(enable, ref, est_state,areaOfInterestCorner)
references_NED = zeros(3,1);
est_state_NED  = zeros(3,1);
phi = est_state(4);
th  = est_state(5);
psi = est_state(6);
coder.extrinsic('evalin','wgs84Ellipsoid','geodetic2ned')    % Reference spheroid
orig = [areaOfInterestCorner(1)   areaOfInterestCorner(2)   areaOfInterestCorner(3)]'; %origine terna NED
wgs84 = wgs84Ellipsoid;
% Cambiamento di riferimento da WGS84 a NED frame
if enable == 1
   [x_ref, y_ref, z_ref] = geodetic2ned(ref(1),ref(2),ref(3),orig(1),orig(2),orig(3),wgs84);
   references_NED = [x_ref, y_ref, z_ref]';
   [x_est, y_est, z_est] = geodetic2ned(est_state(1),est_state(2),est_state(3),orig(1),orig(2),orig(3),wgs84);
   est_state_NED  = [x_est, y_est, est_state(3)]';
   % Calcolo errore posizione da NED a BODY frame
   err_NED  = references_NED - est_state_NED;
   R_z_psi = [cos(psi)    sin(psi)     0;
              -sin(psi)   cos(psi)     0;
                 0           0         1];
          
   R_y_th =  [cos(th)        0      -sin(th);
                 0           1         0;
              sin(th)        0       cos(th)];
       
   R_x_phi = [   1           0             0;
                 0         cos(phi)    sin(phi);
                 0        -sin(phi)    cos(phi)];
          
   R_NB = ((R_z_psi')*(R_y_th')*(R_x_phi'))';
   err_pos_BODY = R_NB * err_NED;
   err_pos = err_pos_BODY(2);
else
   err_pos = 0;
end
end

== matlab function TeamA_PAsqualo1/Controller/diving controller/sway_controller/Sway PID controller/compute_velocity_error ==
  settings: updateMethod=DISCRETE  sampleTime=0.1
  data: enable input size=1; err_vel output size=1; v_des input size=1; est_meas input size=[12 1]
function err_vel = fcn(enable,v_des,est_meas)
if enable == 1
   err_vel =  v_des - est_meas(8);
else
    err_vel = 0;
end
end

== matlab function TeamA_PAsqualo1/Controller/diving controller/yaw_controller/Yaw PID controller/compute_orientation_errors ==
  settings: updateMethod=DISCRETE  sampleTime=0.1
  data: enable input size=1; err_orient output size=1; ref input size=[12 1]; est_state input size=[12 1]
function err_orient = fcn(enable, ref, est_state)
coder.extrinsic('wrapToPi');
err_orient = 0;
phi = est_state(4);
th  = est_state(5);
%
J_inv = [1       0          -sin(th); 
         0   cos(phi)  cos(th)*sin(phi);
         0  -sin(phi)  cos(th)*cos(phi)];
if enable == 1
   err_orient_1 = wrapToPi(J_inv*([ref(4);ref(5);ref(6)] -...
                           [est_state(4);est_state(5);est_state(6)]));
else 
   err_orient_1 = zeros(3,1);
end
err_orient = err_orient_1(3);
end

== matlab function TeamA_PAsqualo1/Controller/diving controller/yaw_controller/Yaw PID controller/compute_velocity_error ==
  data: enable input; err_vel output; v_des input; est_meas input
function err_vel = fcn(enable,v_des,est_meas)
if enable == 1
   err_vel =  v_des - est_meas(12);
else
    err_vel = 0;
end

== matlab function TeamA_PAsqualo1/Controller/positioning controller/heave_controller/Heave PID controller/compute_position_errors ==
  data: enable input; err_pos output; ref input; est_state input; areaOfInterestCorner parameter
function err_pos = fcn(enable, ref, est_state,areaOfInterestCorner)
references_NED = zeros(3,1);
est_state_NED  = zeros(3,1);
phi = est_state(4);
th  = est_state(5);
psi = est_state(6);
coder.extrinsic('evalin','wgs84Ellipsoid','geodetic2ned')    
orig = [areaOfInterestCorner(1)   areaOfInterestCorner(2)   areaOfInterestCorner(3)]'; %origine terna NED
wgs84 = wgs84Ellipsoid;
% Cambiamento di riferimento da WGS84 a NED frame
if enable == 1
   [x_ref, y_ref, z_ref] = geodetic2ned(ref(1),ref(2),ref(3),orig(1),orig(2),orig(3),wgs84);
   references_NED = [x_ref, y_ref, z_ref]';
   [x_est, y_est, z_est] = geodetic2ned(est_state(1),est_state(2),est_state(3),orig(1),orig(2),orig(3),wgs84);
   est_state_NED  =  [x_est, y_est, est_state(3)]';
   % Calcolo errore posizione da NED a BODY frame
   err_NED  = references_NED - est_state_NED;
   R_z_psi = [cos(psi)    sin(psi)     0;
              -sin(psi)   cos(psi)     0;
                 0           0         1];
          
   R_y_th =  [cos(th)        0      -sin(th);
                 0           1         0;
              sin(th)        0       cos(th)];
       
   R_x_phi = [   1           0             0;
                 0         cos(phi)    sin(phi);
                 0        -sin(phi)    cos(phi)];
          
   R_NB = ((R_z_psi')*(R_y_th')*(R_x_phi'))';
   err_pos_BODY = R_NB * err_NED;
   err_pos = err_pos_BODY(3);
else
   err_pos = 0;
end
end

== matlab function TeamA_PAsqualo1/Controller/positioning controller/heave_controller/Heave PID controller/compute_velocity_error ==
  data: enable input; err_vel output; v_des input; est_meas input
function err_vel = fcn(enable,v_des,est_meas)
err_vel = 0;
if enable == 1
   err_vel =  v_des - est_meas(9);
else 
    err_vel = 0;
end
end

== matlab function TeamA_PAsqualo1/Controller/positioning controller/pitch_controller/Pitch PID controller/compute_orientation_errors ==
  data: enable input; err_orient output; ref input; est_state input
function err_orient = fcn(enable, ref, est_state)
coder.extrinsic('wrapToPi');
err_orient = 0;
phi = est_state(4);
th  = est_state(5);
%
J_inv = [1       0          -sin(th); 
         0   cos(phi)  cos(th)*sin(phi);
         0  -sin(phi)  cos(th)*cos(phi)];
if enable == 1
   err_orient_1 = wrapToPi(J_inv*([ref(4);ref(5);ref(6)] -...
                                [est_state(4);est_state(5);est_state(6)]));
else 
   err_orient_1 = zeros(3,1);
end
err_orient = err_orient_1(2);
end

== matlab function TeamA_PAsqualo1/Controller/positioning controller/pitch_controller/Pitch PID controller/compute_velocity_error ==
  data: enable input; err_vel output; v_des input; est_meas input
function err_vel = fcn(enable,v_des,est_meas)
if enable == 1
   err_vel =  v_des - est_meas(11);
else
    err_vel = 0;
end
end

== matlab function TeamA_PAsqualo1/Controller/positioning controller/roll_controller/Roll PID controller/compute_orientation_errors ==
  data: enable input; err_orient output; ref input; est_state input
function err_orient = fcn(enable, ref, est_state)
coder.extrinsic('wrapToPi');
err_orient = 0;
phi = est_state(4);
th  = est_state(5);
%
J_inv = [1       0          -sin(th); 
         0   cos(phi)  cos(th)*sin(phi);
         0  -sin(phi)  cos(th)*cos(phi)];
if enable == 1
   err_orient_1 = wrapToPi(J_inv*([ref(4);ref(5);ref(6)] -...
                           [est_state(4);est_state(5);est_state(6)]));
else 
   err_orient_1 = zeros(3,1);
end
err_orient = err_orient_1(1);
end

== matlab function TeamA_PAsqualo1/Controller/positioning controller/roll_controller/Roll PID controller/compute_velocity_error ==
  data: enable input; err_vel output; v_des input; est_meas input
function err_vel = fcn(enable,v_des,est_meas)
if enable == 1
   err_vel =  v_des - est_meas(10);
else 
    err_vel = 0;
end
end
